simulink model "geki"  (Simulink 8.3)
settings: Solver=ode3  StartTime=0.0  StopTime=1  FixedStep=1e-2  RelTol=1e-3
settings Model: Creator=Administrator  LastModifiedBy=User
settings OptimizationCC: ExpressionDepthLimit=2147483647
settings DebuggingCC: SolverPrmCheckMsg=none  FcnCallInpInsideContextMsg=EnableAllAsWarning  FrameProcessingCompatibilityMsg=error
settings GRTTargetCC: CombineOutputUpdateFcns=on  GRTInterface=off
settings ConfigComp: CovMetricSettings=dw  CovHtmlReporting=on  CovSaveCumulativeToWorkspaceVar=on  CovSaveSingleToWorkspaceVar=on  CovModelRefEnable=Off  CovExternalEMLEnable=off

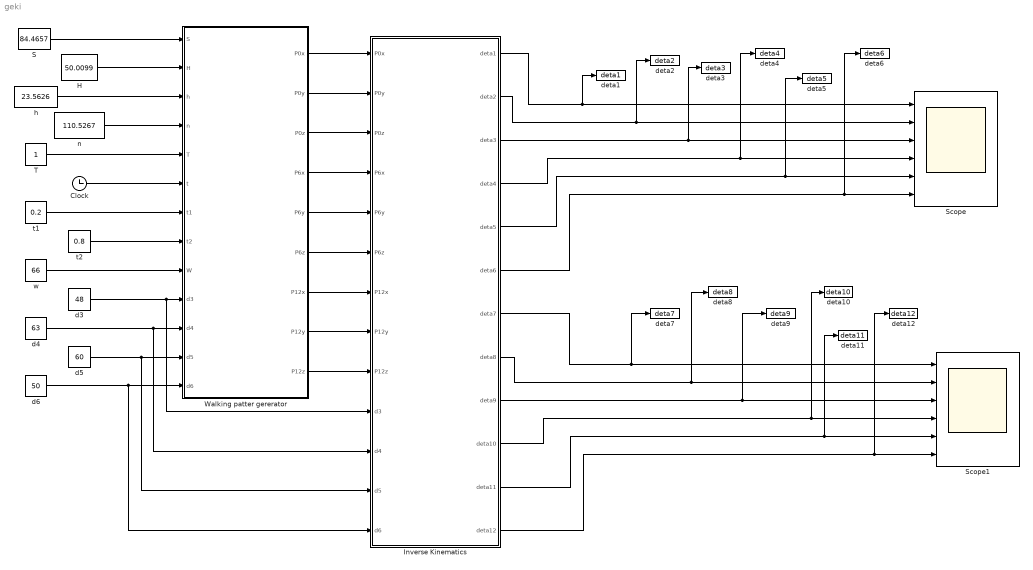
== system geki ==
  Clock : Clock
  H : Constant  Value=50.0099
  Inverse Kinematics : MATLAB Function  TreatAsAtomicUnit=on
  S : Constant  Value=84.4657
  Scope : Scope  NumInputPorts=6
  Scope1 : Scope  NumInputPorts=6
  T : Constant
  Walking patter gererator : MATLAB Function  TreatAsAtomicUnit=on
  d3 : Constant  Value=48
  d4 : Constant  Value=63
  d5 : Constant  Value=60
  d6 : Constant  Value=50
  deta1 : ToWorkspace  VariableName=deta1  SampleTime=-1
  deta10 : ToWorkspace  VariableName=deta10  SampleTime=-1
  deta11 : ToWorkspace  VariableName=deta11  SampleTime=-1
  deta12 : ToWorkspace  VariableName=deta12  SampleTime=-1
  deta2 : ToWorkspace  VariableName=deta2  SampleTime=-1
  deta3 : ToWorkspace  VariableName=deta3  SampleTime=-1
  deta4 : ToWorkspace  VariableName=deta4  SampleTime=-1
  deta5 : ToWorkspace  VariableName=deta5  SampleTime=-1
  deta6 : ToWorkspace  VariableName=deta6  SampleTime=-1
  deta7 : ToWorkspace  VariableName=deta7  SampleTime=-1
  deta8 : ToWorkspace  VariableName=deta8  SampleTime=-1
  deta9 : ToWorkspace  VariableName=deta9  SampleTime=-1
  h : Constant  Value=23.5626
  n : Constant  Value=110.5267
  t1 : Constant  Value=0.2
  t2 : Constant  Value=0.8
  w : Constant  Value=66
  wires:
  H/1 -> Walking patter gererator/2(H)
  h/1 -> Walking patter gererator/3(h)
  n/1 -> Walking patter gererator/4(n)
  w/1 -> Walking patter gererator/9(W)
  S/1 -> Walking patter gererator/1(S)
  t1/1 -> Walking patter gererator/7(t1)
  t2/1 -> Walking patter gererator/8(t2)
  d4/1 -> Inverse Kinematics/11(d4), Walking patter gererator/11(d4)
  d5/1 -> Inverse Kinematics/12(d5), Walking patter gererator/12(d5)
  d6/1 -> Inverse Kinematics/13(d6), Walking patter gererator/13(d6)
  d3/1 -> Inverse Kinematics/10(d3), Walking patter gererator/10(d3)
  T/1 -> Walking patter gererator/5(T)
  Clock/1 -> Walking patter gererator/6(t)
  Walking patter gererator/1(P0x) -> Inverse Kinematics/1(P0x)
  Walking patter gererator/2(P0y) -> Inverse Kinematics/2(P0y)
  Walking patter gererator/3(P0z) -> Inverse Kinematics/3(P0z)
  Walking patter gererator/4(P6x) -> Inverse Kinematics/4(P6x)
  Walking patter gererator/5(P6y) -> Inverse Kinematics/5(P6y)
  Walking patter gererator/6(P6z) -> Inverse Kinematics/6(P6z)
  Walking patter gererator/7(P12x) -> Inverse Kinematics/7(P12x)
  Walking patter gererator/8(P12y) -> Inverse Kinematics/8(P12y)
  Walking patter gererator/9(P12z) -> Inverse Kinematics/9(P12z)
  Inverse Kinematics/1(deta1) -> deta1/1, Scope/1
  Inverse Kinematics/2(deta2) -> deta2/1, Scope/2
  Inverse Kinematics/3(deta3) -> deta3/1, Scope/3
  Inverse Kinematics/4(deta4) -> deta4/1, Scope/4
  Inverse Kinematics/5(deta5) -> deta5/1, Scope/5
  Inverse Kinematics/6(deta6) -> deta6/1, Scope/6
  Inverse Kinematics/7(deta7) -> deta7/1, Scope1/1
  Inverse Kinematics/8(deta8) -> deta8/1, Scope1/2
  Inverse Kinematics/9(deta9) -> deta9/1, Scope1/3
  Inverse Kinematics/10(deta10) -> deta10/1, Scope1/4
  Inverse Kinematics/11(deta11) -> deta11/1, Scope1/5
  Inverse Kinematics/12(deta12) -> deta12/1, Scope1/6

== matlab function Inverse Kinematics ==
  data: deta1 output double; deta2 output double; P0x input double; P0y input double; P0z input double; P6x input double; P6y input double; deta3 output double; P6z input double; P12x input double; P12y input double; P12z input double; deta4 output double; deta5 output double; deta6 output double; deta7 output double; deta8 output double; deta9 output double; deta10 output double; deta11 output double; deta12 output double; d3 input double; d4 input double; d5 input double; d6 input double
function [deta1,deta2,deta3,deta4,deta5,deta6,deta7,deta8,deta9,deta10,deta11,deta12] = fcn(P0x,P0y,P0z,P6x,P6y,P6z,P12x,P12y,P12z,d3,d4,d5,d6)
x_l=P0x-P6x;
y_l=-P6y;
z_l=P0z-P6z;
x_r=P12x-P6x;
y_r=-P6y;
z_r=P12z-P6z;
l_l=sqrt(x_l*x_l+0.25*y_l*y_l+(z_l+d3+d6)*(z_l+d3+d6));
l_r=sqrt(x_r*x_r+0.25*y_r*y_r+(z_r+d3+d6)*(z_r+d3+d6));
detaA=acos((d4*d4+d5*d5-l_l*l_l)/(2*d4*d5));
detaB=acos(d4*sin(detaA)/l_l);
detaC=acos((d4*d4+d5*d5-l_r*l_r)/(2*d4*d5));
detaD=acos(d4*sin(detaC)/l_r);
deta1=atan(y_l/z_l);
deta6=deta1;
deta5=pi/2 - detaA + detaB + asin(x_l/l_l);
deta3=pi-detaA;
deta2=(deta3 - deta5);
deta10=pi-detaC;
deta8=pi/2 - detaC + detaD + asin(x_r/l_r);
deta12=atan(y_r/z_r);
deta7=deta12;
deta11=(deta10 - deta8);
deta4=0;
deta9=0;
end

== matlab function Walking patter gererator ==
  data: P0x output double; P0y output double; S input double; H input double; h input double; n input double; T input double; P0z output double; t input double; t1 input double; t2 input double; W input double; d3 input double; d4 input double; d5 input double; d6 input double; P6x output double; P6y output double; P6z output double; P12x output double; P12y output double; P12z output double
function [P0x,P0y,P0z,P6x,P6y,P6z,P12x,P12y,P12z] = fcn(S,H,h,n,T,t,t1,t2,W,d3,d4,d5,d6)
P0x=0;
P0y=0;
P0z=0;
P12x=(S/2)*sin(pi*(t-T/2)/T);
P12y=-W;
P12z=H*sin(pi*((P12x/S)+0.5));
P6x=(S/4)*sin((pi/T)*(tt(t,T)-T/2));
P6y=n*sin(pi/(2*t1)*tt(t,T))*(u(tt(t,T))-u(tt(t,T)-t1))...
+n*(u(tt(t,T)-t1)-u(tt(t,T)-t2))...
+n*cos(pi/(2*(T-t2))*(tt(t,T)-t2))*(u(tt(t,T)-t2)-u(tt(t,T)-T));
P6z=d3+d4+d5+d6-h;
end
function to = tt(t,T)
    if (t>=0 && t<=T)
        to=t;
    else
       to=t-T;
    end
end
%%%%%%%
%%% P6y
function ti=u(t)
    if (t>=0)
        ti=1;
    else
        ti=0;
    end
end
